simulink model "SiL_gram"  (R2025b)
settings: Solver=ode2  StartTime=0.0  StopTime=t_end  FixedStep=1/400  RelTol=1e-3
PreLoadFcn:
  | stepsize_sim = evalin('base', get_param(bdroot, 'FixedStep'));
undefined symbols (not defined in the file or in its folder): defaultConsts, defaultWP, DiscIntNeverNeededParam, dspblkCoreblockFVToolHelper, gcbh, navConsts, sensors, stepsize_ctrl
libraries: simulink x7, sharedutil x1, sharedtransform x1, aerolibanimutils x1
(part 3 of 3)

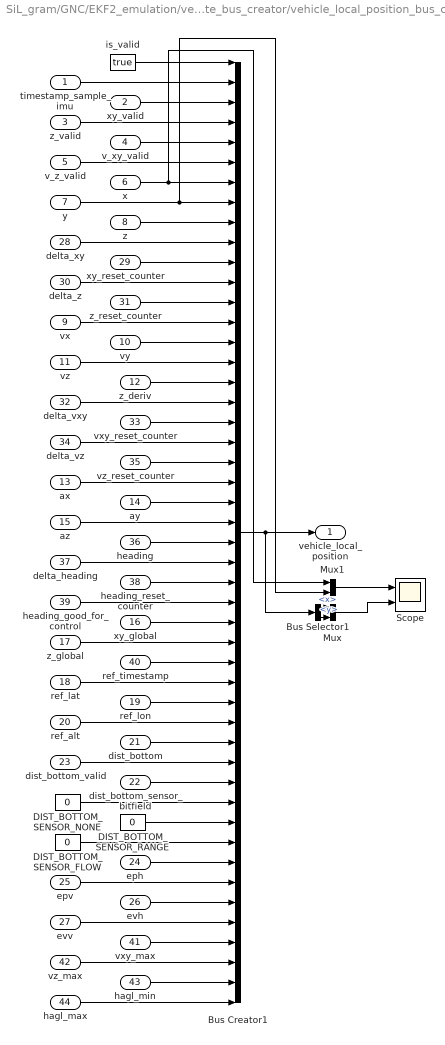
== system SiL_gram/GNC/EKF2_emulation/vehicle_state_bus_creator/vehicle_local_position_bus_creator ==
  timestamp_sample_imu : Inport
  xy_valid : Inport  Port=2  OutDataTypeStr=boolean  PortDimensions=1
  z_valid : Inport  Port=3  OutDataTypeStr=boolean  PortDimensions=1
  v_xy_valid : Inport  Port=4  OutDataTypeStr=boolean  PortDimensions=1
  v_z_valid : Inport  Port=5  OutDataTypeStr=boolean  PortDimensions=1
  x : Inport  Port=6  OutDataTypeStr=single  PortDimensions=1
  y : Inport  Port=7  OutDataTypeStr=single  PortDimensions=1
  z : Inport  Port=8  OutDataTypeStr=single  PortDimensions=1
  vx : Inport  Port=9  OutDataTypeStr=single  PortDimensions=1
  vy : Inport  Port=10  OutDataTypeStr=single  PortDimensions=1
  vz : Inport  Port=11  OutDataTypeStr=single  PortDimensions=1
  z_deriv : Inport  Port=12  OutDataTypeStr=single  PortDimensions=1
  ax : Inport  Port=13  OutDataTypeStr=single  PortDimensions=1
  ay : Inport  Port=14  OutDataTypeStr=single  PortDimensions=1
  az : Inport  Port=15  OutDataTypeStr=single  PortDimensions=1
  xy_global : Inport  Port=16  OutDataTypeStr=boolean  PortDimensions=1
  z_global : Inport  Port=17  OutDataTypeStr=boolean  PortDimensions=1
  ref_lat : Inport  Port=18  OutDataTypeStr=double  PortDimensions=1
  ref_lon : Inport  Port=19  OutDataTypeStr=double  PortDimensions=1
  ref_alt : Inport  Port=20  OutDataTypeStr=single  PortDimensions=1
  dist_bottom : Inport  Port=21  OutDataTypeStr=single  PortDimensions=1
  dist_bottom_sensor_bitfield : Inport  Port=22  OutDataTypeStr=uint8  PortDimensions=1
  dist_bottom_valid : Inport  Port=23  OutDataTypeStr=boolean  PortDimensions=1
  eph : Inport  Port=24  OutDataTypeStr=single  PortDimensions=1
  epv : Inport  Port=25  OutDataTypeStr=single  PortDimensions=1
  evh : Inport  Port=26  OutDataTypeStr=single  PortDimensions=1
  evv : Inport  Port=27  OutDataTypeStr=single  PortDimensions=1
  delta_xy : Inport  Port=28  OutDataTypeStr=single  PortDimensions=2
  xy_reset_counter : Inport  Port=29  OutDataTypeStr=uint8  PortDimensions=1
  delta_z : Inport  Port=30  OutDataTypeStr=single  PortDimensions=1
  z_reset_counter : Inport  Port=31  OutDataTypeStr=uint8  PortDimensions=1
  delta_vxy : Inport  Port=32  OutDataTypeStr=single  PortDimensions=2
  vxy_reset_counter : Inport  Port=33  OutDataTypeStr=uint8  PortDimensions=1
  delta_vz : Inport  Port=34  OutDataTypeStr=single  PortDimensions=1
  vz_reset_counter : Inport  Port=35  OutDataTypeStr=uint8  PortDimensions=1
  heading : Inport  Port=36  OutDataTypeStr=single  PortDimensions=1
  delta_heading : Inport  Port=37  OutDataTypeStr=single  PortDimensions=1
  heading_reset_counter : Inport  Port=38  OutDataTypeStr=uint8  PortDimensions=1
  heading_good_for_control : Inport  Port=39  OutDataTypeStr=boolean  PortDimensions=1
  ref_timestamp : Inport  Port=40  OutDataTypeStr=double  PortDimensions=1
  vxy_max : Inport  Port=41  OutDataTypeStr=single  PortDimensions=1
  vz_max : Inport  Port=42  OutDataTypeStr=single  PortDimensions=1
  hagl_min : Inport  Port=43  OutDataTypeStr=single  PortDimensions=1
  hagl_max : Inport  Port=44  OutDataTypeStr=single  PortDimensions=1
  Bus Selector1 : BusSelector  OutputSignals=x,y
  Bus Creator1 : BusCreator  Inputs=48  OutDataTypeStr=Bus: vehicle_local_position_bus
      settings: InheritFromInputs=off
  DIST_BOTTOM_SENSOR_FLOW : Constant  Value=0  OutDataTypeStr=uint8
  DIST_BOTTOM_SENSOR_NONE : Constant  Value=0  OutDataTypeStr=uint8
  DIST_BOTTOM_SENSOR_RANGE : Constant  Value=0  OutDataTypeStr=uint8
  Mux : Mux  Inputs=2
  Mux1 : Mux  Inputs=2
  Scope : Scope  NumInputPorts=2
      settings: ActiveDisplayYMinimum=-586.90811681747437  ActiveDisplayYMaximum=109.35261678695677  DataLoggingVariableName=ScopeData7
  is_valid : Constant  Value=true  OutDataTypeStr=boolean
  vehicle_local_position : Outport  OutDataTypeStr=Bus: vehicle_local_position_bus  VectorParamsAs1DForOutWhenUnconnected=off
  wires:
  is_valid/1 -> Bus Creator1/1
  xy_valid/1 -> Bus Creator1/3
  z_valid/1 -> Bus Creator1/4
  v_xy_valid/1 -> Bus Creator1/5
  v_z_valid/1 -> Bus Creator1/6
  x/1 -> Mux1/1, Bus Creator1/7
  y/1 -> Mux1/2, Bus Creator1/8
  z/1 -> Bus Creator1/9
  delta_xy/1 -> Bus Creator1/10
  xy_reset_counter/1 -> Bus Creator1/11
  delta_z/1 -> Bus Creator1/12
  z_reset_counter/1 -> Bus Creator1/13
  vx/1 -> Bus Creator1/14
  vy/1 -> Bus Creator1/15
  vz/1 -> Bus Creator1/16
  z_deriv/1 -> Bus Creator1/17
  delta_vxy/1 -> Bus Creator1/18
  vxy_reset_counter/1 -> Bus Creator1/19
  delta_vz/1 -> Bus Creator1/20
  vz_reset_counter/1 -> Bus Creator1/21
  ax/1 -> Bus Creator1/22
  ay/1 -> Bus Creator1/23
  az/1 -> Bus Creator1/24
  heading/1 -> Bus Creator1/25
  xy_global/1 -> Bus Creator1/29
  z_global/1 -> Bus Creator1/30
  ref_timestamp/1 -> Bus Creator1/31
  ref_lat/1 -> Bus Creator1/32
  ref_lon/1 -> Bus Creator1/33
  ref_alt/1 -> Bus Creator1/34
  dist_bottom/1 -> Bus Creator1/35
  dist_bottom_sensor_bitfield/1 -> Bus Creator1/37
  dist_bottom_valid/1 -> Bus Creator1/36
  eph/1 -> Bus Creator1/41
  epv/1 -> Bus Creator1/42
  evh/1 -> Bus Creator1/43
  evv/1 -> Bus Creator1/44
  vxy_max/1 -> Bus Creator1/45
  vz_max/1 -> Bus Creator1/46
  hagl_min/1 -> Bus Creator1/47
  hagl_max/1 -> Bus Creator1/48
  Bus Creator1/1 -> Bus Selector1/1, vehicle_local_position/1
  timestamp_sample_imu/1 -> Bus Creator1/2
  heading_good_for_control/1 -> Bus Creator1/28
  heading_reset_counter/1 -> Bus Creator1/27
  delta_heading/1 -> Bus Creator1/26
  DIST_BOTTOM_SENSOR_NONE/1 -> Bus Creator1/38
  DIST_BOTTOM_SENSOR_FLOW/1 -> Bus Creator1/40
  DIST_BOTTOM_SENSOR_RANGE/1 -> Bus Creator1/39
  Bus Selector1/1 -> Mux/1  "<x>"
  Bus Selector1/2 -> Mux/2  "<y>"
  Mux/1 -> Scope/2
  Mux1/1 -> Scope/1

== system SiL_gram/GNC/mavlink_receiver.cpp/GPS/Subsystem ==
  n : Inport
  e : Inport  Port=2
  d : Inport  Port=3
  Sqrt : Sqrt
  Square : Math  Operator=square
  Square1 : Math  Operator=square
  Square2 : Math  Operator=square
  Sum : Sum  Inputs=+++
  Out1 : Outport
  wires:
  Sqrt/1 -> Out1/1
  Sum/1 -> Sqrt/1
  n/1 -> Square/1
  Square/1 -> Sum/1
  d/1 -> Square2/1
  e/1 -> Square1/1
  Square1/1 -> Sum/2
  Square2/1 -> Sum/3

== system SiL_gram/GNC/mavlink_receiver.cpp/Waypoints/switch WPs ==
  Constant : Constant  Value=defaultWP.flightplan
  Manual Switch : ManualSwitch  CurrentSetting=0
  Terminator : Terminator
  landing WP : MATLAB Function  TreatAsAtomicUnit=on
  new flightplan : MATLAB Function  TreatAsAtomicUnit=on
  original : Outport
  modified : Outport  Port=2
  wires:
  new flightplan/1(flt_new) -> Manual Switch/1
  Constant/1 -> original/1, Manual Switch/2, new flightplan/1(fltplan)
  Manual Switch/1 -> modified/1
  landing WP/1(flt_new) -> Terminator/1

== matlab function SiL_gram/GNC/EKF2_emulation/MATLAB Function ==
  data: quat input single; eul_rad output single
function eul_rad=quat2euler(quat)

eul_rad = single([0;0;0]);
ysqr = quat(3) * quat(3);

t0 = 2 * (quat(1) * quat(2) + quat(3) * quat(4));
t1 = 1 - 2 * (quat(2) * quat(2) + ysqr);
eul_rad(1) = atan2(t0, t1);

t2 = 2 * (quat(1) * quat(3) - quat(4) * quat(2));
if t2 > 1
    t2 = single(1);
elseif t2 < -1
    t2 = -single(1);
end
eul_rad(2) = asin(t2);

t3 = 2 * (quat(1) * quat(4) + quat(2) * quat(3));
t4 = 1 - 2 * (ysqr + quat(4) * quat(4));
eul_rad(3) = atan2(t3, t4);

end

== matlab function SiL_gram/GNC/EKF2_emulation/MATLAB Function1 ==
  data: baro_rel input Bus: ifr_baro; h_ref input; ref_pos input; ref_valid input; baro_abs output Bus: ifr_baro
function baro_abs  = fcn(baro_rel,h_ref,ref_pos,ref_valid)

baro_abs.isValid = baro_rel.isValid;

if ref_valid
    baro_abs.height  = baro_rel.height + single(ref_pos(3)*1e-3);
else
    baro_abs.height  = baro_rel.height + h_ref;
end

end

== matlab function SiL_gram/GNC/mavlink_receiver.cpp/ifr_imu_filter.cpp/filterAccelMeasurementSecondOrder ==
  data: ome input; y output; zet input; acc input; stepsize_sim parameter
function y = fcn(ome,zet,acc,stepsize_sim)
persistent ykm1 ykm2 ukm1 ukm2

if isempty(ykm1)
    ykm1 = zeros(3,1,'single');
    ykm2 = zeros(3,1,'single');
    ukm1 = zeros(3,1,'single');
    ukm2 = zeros(3,1,'single');
end

subs1 = zet*ome*stepsize_sim;
subs2 = ome^2*stepsize_sim^2;

num = ykm2*(4*subs1-subs2-4) + ykm1*(8-2*subs2) + (ukm2+2*ukm1+acc)*subs2;
den = (4*subs1+subs2+4);

yk = num/den;
ukm2 = ukm1;
ukm1 = acc;
ykm2 = ykm1;
ykm1 = yk;

y = yk;

== matlab function SiL_gram/GNC/mavlink_receiver.cpp/Waypoints/switch WPs/new flightplan ==
  data: fltplan input; flt_new output
function flt_new = fcn(fltplan)

flt_new = fltplan;
flt_new(1,1)=5;
flt_new(6,:)=[-400,150,-100];
%flt_new(:,2)=flt_new(:,2)+200;
flt_new(:,3)=flt_new(:,3)-60;
flt_new(5,3)=flt_new(5,3)+20;

== matlab function SiL_gram/Sensors/ifr_imu_filter.cpp/MATLAB Function ==
  data: filt_num output single; filt_den output single; zeta input single; diff_num output single; diff_den output single; omega input single
function [filt_num,filt_den,diff_num,diff_den]  = tbv(zeta,omega)

T = single(0.01);
w = omega;
z = zeta;

scale = T^2*w^2+4*T*w*z+4;

%Discrete time IMU derivative and second order washout filter transfer function. See filter_design.m for more details.
diff_num = [2*T*w^2 0 -2*T*w^2]/scale;
diff_den = [T^2*w^2+4*T*w*z+4 2*T^2*w^2-8 T^2*w^2-4*T*w*z+4]/scale;

%Discrete time second order washout filter to synchronize phase shift between IMU derivative and actuator position signals. See filter_design.m for more details.
filt_num = [T^2*w^2, 2*T^2*w^2, T^2*w^2]/scale;
filt_den = [T^2*w^2+4*T*w*z+4 2*T^2*w^2-8 T^2*w^2-4*T*w*z+4]/scale;

== matlab function SiL_gram/GNC/mavlink_receiver.cpp/Waypoints/switch WPs/landing WP ==
  data: flt_new output
function flt_new = fcn()

flt_new = zeros(21,3);
flt_new(1,1)=1;
flt_new(2,:)=[100,0,0];

== matlab function SiL_gram/GNC/mavlink_receiver.cpp/ifr_imu_filter.cpp/MATLAB Function ==
  data: filt_num output single; filt_den output single; zeta input single; diff_num output single; diff_den output single; omega input single
function [filt_num,filt_den,diff_num,diff_den]  = tbv(zeta,omega)

T = single(0.01);
w = omega;
z = zeta;

scale = T^2*w^2+4*T*w*z+4;

%Discrete time IMU derivative and second order washout filter transfer function. See filter_design.m for more details.
diff_num = [2*T*w^2 0 -2*T*w^2]/scale;
diff_den = [T^2*w^2+4*T*w*z+4 2*T^2*w^2-8 T^2*w^2-4*T*w*z+4]/scale;

%Discrete time second order washout filter to synchronize phase shift between IMU derivative and actuator position signals. See filter_design.m for more details.
filt_num = [T^2*w^2, 2*T^2*w^2, T^2*w^2]/scale;
filt_den = [T^2*w^2+4*T*w*z+4 2*T^2*w^2-8 T^2*w^2-4*T*w*z+4]/scale;

== matlab function SiL_gram/GNC/mavlink_receiver.cpp/ifr_imu_filter.cpp/filterGyroMeasurementSecondOrder ==
  data: ome input; y output; zet input; rte input; stepsize_sim parameter
function y = fcn(ome,zet,rte,stepsize_sim)
persistent ykm1 ykm2 ukm1 ukm2

if isempty(ykm1)
    ykm1 = zeros(3,1,'single');
    ykm2 = zeros(3,1,'single');
    ukm1 = zeros(3,1,'single');
    ukm2 = zeros(3,1,'single');
end

subs1 = zet*ome*stepsize_sim;
subs2 = ome^2*stepsize_sim^2;

num = ykm2*(4*subs1-subs2-4) + ykm1*(8-2*subs2) + (ukm2+2*ukm1+rte)*subs2;
den = (4*subs1+subs2+4);

yk = num/den;
ukm2 = ukm1;
ukm1 = rte;
ykm2 = ykm1;
ykm1 = yk;

y = yk;

== matlab function SiL_gram/GNC/mavlink_receiver.cpp/ifr_imu_filter.cpp/filterGyroDerivativeSecondOrder ==
  data: ome input; y output; zet input; rte input; stepsize_sim parameter
function y = fcn(ome,zet,rte,stepsize_sim)
persistent ykm1 ykm2 ukm1 ukm2

if isempty(ykm1)
    ykm1 = zeros(3,1,'single');
    ykm2 = zeros(3,1,'single');
    ukm1 = zeros(3,1,'single');
    ukm2 = zeros(3,1,'single');
end

subs1 = zet*ome*stepsize_sim;
subs2 = ome^2*stepsize_sim^2;

num = ykm2*(4*subs1-subs2-4) + ykm1*(8-2*subs2) + 2*(rte-ukm2)*ome^2*stepsize_sim;
den = (4*subs1+subs2+4);

yk = num/den;
ukm2 = ukm1;
ukm1 = rte;
ykm2 = ykm1;
ykm1 = yk;

y = yk;

== matlab function SiL_gram/Sensors/ifr_imu_filter.cpp/filterAccelMeasurementSecondOrder ==
  data: ome input; y output; zet input; acc input; stepsize_sim parameter
function y = fcn(ome,zet,acc,stepsize_sim)
persistent ykm1 ykm2 ukm1 ukm2

if isempty(ykm1)
    ykm1 = zeros(3,1,'single');
    ykm2 = zeros(3,1,'single');
    ukm1 = zeros(3,1,'single');
    ukm2 = zeros(3,1,'single');
end

subs1 = zet*ome*stepsize_sim;
subs2 = ome^2*stepsize_sim^2;

num = ykm2*(4*subs1-subs2-4) + ykm1*(8-2*subs2) + (ukm2+2*ukm1+acc)*subs2;
den = (4*subs1+subs2+4);

yk = num/den;
ukm2 = ukm1;
ukm1 = acc;
ykm2 = ykm1;
ykm1 = yk;

y = yk;

== matlab function SiL_gram/Sensors/ifr_imu_filter.cpp/filterGyroDerivativeSecondOrder ==
  data: ome input; y output; zet input; rte input; stepsize_sim parameter
function y = fcn(ome,zet,rte,stepsize_sim)
persistent ykm1 ykm2 ukm1 ukm2

if isempty(ykm1)
    ykm1 = zeros(3,1,'single');
    ykm2 = zeros(3,1,'single');
    ukm1 = zeros(3,1,'single');
    ukm2 = zeros(3,1,'single');
end

subs1 = zet*ome*stepsize_sim;
subs2 = ome^2*stepsize_sim^2;

num = ykm2*(4*subs1-subs2-4) + ykm1*(8-2*subs2) + 2*(rte-ukm2)*ome^2*stepsize_sim;
den = (4*subs1+subs2+4);

yk = num/den;
ukm2 = ukm1;
ukm1 = rte;
ykm2 = ykm1;
ykm1 = yk;

y = yk;

== matlab function SiL_gram/Sensors/ifr_imu_filter.cpp/filterGyroMeasurementSecondOrder ==
  data: ome input; y output; zet input; rte input; stepsize_sim parameter
function y = fcn(ome,zet,rte,stepsize_sim)
persistent ykm1 ykm2 ukm1 ukm2

if isempty(ykm1)
    ykm1 = zeros(3,1,'single');
    ykm2 = zeros(3,1,'single');
    ukm1 = zeros(3,1,'single');
    ukm2 = zeros(3,1,'single');
end

subs1 = zet*ome*stepsize_sim;
subs2 = ome^2*stepsize_sim^2;

num = ykm2*(4*subs1-subs2-4) + ykm1*(8-2*subs2) + (ukm2+2*ukm1+rte)*subs2;
den = (4*subs1+subs2+4);

yk = num/den;
ukm2 = ukm1;
ukm1 = rte;
ykm2 = ykm1;
ykm1 = yk;

y = yk;

== matlab function SiL_gram/GNC/mavlink_receiver.cpp/Waypoints/MATLAB Function2 ==
  data: refPos input; llh2ned input; flightplan input; wp_lla output Bus: waypoint_list_bus
function wp_lla = mat2bus(refPos,llh2ned, flightplan)

wp_lla.is_valid = true;
wp_lla.lat = (single(refPos(1))+flightplan(2:end,1)/llh2ned(1))/1e7; %north
wp_lla.lon = (single(refPos(2))+flightplan(2:end,2)/llh2ned(2))/1e7; %east
wp_lla.alt = flightplan(2:end,3)/llh2ned(3)/1e3; %down
wp_lla.count = uint16(flightplan(1,1));

end

== matlab function SiL_gram/Sensors/ifr_imu_filter.cpp/IMU/Placement outside COG ==
  data: omega input; centrifugal_acc output; lever input; dwdt input
function centrifugal_acc = fcn(omega, lever, dwdt)

%centrifugal acceleration is -omega x(omega x lever)
centrifugal_acc = zeros(3,1);
centrifugal_acc = cross(omega,cross(omega,lever)) + cross(dwdt, lever);

== matlab function SiL_gram/GNC/EKF2_emulation/MATLAB Function8 ==
  data: gyro_raw input Bus: sensor_gyro_bus; gyro_m output; acc_raw input Bus: sensor_accel_bus; acc_m output; imu_filter input Bus: ifr_imu_filtered_bus; param input Bus: nav_parameterBus
function [gyro_m,acc_m] = fcn(gyro_raw,acc_raw,imu_filter,param)
pix_orientation = [param.pix_roll;param.pix_pitch;param.pix_yaw];

T1 = [1 0 0;0 cos(pix_orientation(1)) sin(pix_orientation(1));0 -sin(pix_orientation(1)) cos(pix_orientation(1))];
T2 = [cos(pix_orientation(2)) 0 -sin(pix_orientation(2));0 1 0;sin(pix_orientation(2)) 0 cos(pix_orientation(2))];
T3 = [cos(pix_orientation(3)) sin(pix_orientation(3)) 0;-sin(pix_orientation(3)) cos(pix_orientation(3)) 0;0 0 1];
T = T1*T2*T3;

if isequal(param.imu_filt.use_acc,single(1))
    acc_m = imu_filter.acc_filt;
else
    acc_m = T*[acc_raw.x;acc_raw.y;acc_raw.z];
end

if isequal(param.imu_filt.use_rte,single(1))
    gyro_m = imu_filter.rates_filt;
else
    gyro_m = T*[gyro_raw.x;gyro_raw.y;gyro_raw.z];
end

== matlab function SiL_gram/Remote_Control/MATLAB Function ==
  data: cur input; prev input; val input; y output
function y = add(cur,prev,val)

if isequal(prev,0)
    y = val + cur;
else
    y = val;
end

== matlab function SiL_gram/Remote_Control/MATLAB Function1 ==
  data: cur input; prev input; val input; y output
function y = add(cur,prev,val)

if isequal(prev,0)
    y = val + cur;
else
    y = val;
end

== matlab function SiL_gram/GNC/EKF2_emulation/acc transformation4 ==
  data: acc_b input; euler input; acc_g output; navConsts parameter Bus: nav_constantsBus
function acc_g  = acc_transform(acc_b,euler,navConsts)

tf3 = [cos(-euler(3)) sin(-euler(3)) 0; -sin(-euler(3)) cos(-euler(3)) 0; 0 0 1];
tf2 = [cos(-euler(2)) 0 -sin(-euler(2)); 0 1 0; sin(-euler(2)) 0 cos(-euler(2))];
tf1 = [1 0 0; 0 cos(-euler(1)) sin(-euler(1)); 0 -sin(-euler(1)) cos(-euler(1))];

acc_g = tf3*tf2*tf1*(acc_b)+[0;0;navConsts.g];

== matlab function SiL_gram/GNC/EKF2_emulation/barometer preprocessor ==
  settings: updateMethod=DISCRETE
  data: rawBaroData input Bus: sensor_baro_bus size=1; analysisParams output; height output; params input Bus: nav_parameterBus size=1; fixReference input boolean size=1; baro_rel output Bus: ifr_baro size=1; height_ref output; navConsts parameter
function [analysisParams,height,baro_rel,height_ref] = preprocessBaro(rawBaroData,params,fixReference,navConsts)
persistent refHeight_dyn fixed
if params.dynRefHeight
    loopIdentifier = single(1);
    if isempty(refHeight_dyn)
        refHeight_dyn = single(navConsts.initialPositionLla(3));
        fixed=false;
        loopIdentifier = single(10);
    end
    if isempty(fixed)
        fixed=false;
        loopIdentifier = loopIdentifier+single(100);
    end
    
    baro_rel.isValid=(rawBaroData.is_valid && rawBaroData.pressure>500);
    height=computeHeightFromPressure(rawBaroData.pressure, navConsts);
    if ~fixed
        loopIdentifier = loopIdentifier+single(1000);
        baro_rel.height=single(0);
        if fixReference
            fixed=true;
        else
            if navConsts.airStart %air start in simulation
            else
                refHeight_dyn = refHeight_dyn+params.biasSmoothingGain*(height-refHeight_dyn);
                loopIdentifier = loopIdentifier+single(10000);
            end
        end
    else
        baro_rel.height=height-refHeight_dyn;
        %baro.height=height;
    end
    height_ref = refHeight_dyn;
else
    loopIdentifier = single(0);
    refHeight_stat = params.referenceHeight;
    baro_rel.isValid=(rawBaroData.is_valid && rawBaroData.pressure>500);
    height=computeHeightFromPressure(rawBaroData.pressure, navConsts);
    if fixReference
        baro_rel.height=single(0);
    else
        baro_rel.height=height-refHeight_stat;
        %baro.height=height;
    end
    height_ref = refHeight_stat;
end
analysisParams = [navConsts.initialPositionLla(3),height,height_ref,loopIdentifier];
end

function height=computeHeightFromPressure(pressure, constants)
height=constants.referenceTemperature/constants.temperatureGradient*(1-(pressure/constants.referencePressure)^((constants.atmosphereKappa-1)/constants.atmosphereKappa));
end

== matlab function SiL_gram/GNC/EKF2_emulation/delay compensation ==
  data: translation input single size=6; position output single size=3; attitude output single size=4; rotation input single size=4; delRot input single size=4; delPos input single size=3; delVel input single size=3; delAtt input single size=4; velocity output single size=3; navConsts parameter size=1
function [position, attitude, velocity] = fcn(translation,rotation,delRot,delPos,delVel,delAtt,navConsts)
    timeDelay=navConsts.filterDelay;
    
    geoToRef=quaternionProduct(delAtt, [delRot(1); -delRot(2:4)]);
    refToGeoMat=quatToMat(geoToRef)';
    position=delPos+timeDelay*delVel+refToGeoMat*translation(1:3)+0.5*timeDelay^2*[0; 0; navConsts.g];
    velocity=delVel+refToGeoMat*translation(4:6)+timeDelay*[0; 0; navConsts.g];
    attitude=quaternionProduct(geoToRef, rotation);
end

function prod=quaternionProduct(q, p)
    [q0, qVec, p0, pVec]=deal(q(1), q(2:4), p(1), p(2:4));
    prod=[q0*p0-qVec'*pVec; q0*pVec+p0*qVec+cross(qVec, pVec)];
end

function mat=quatToMat(quat)
    [q0, q1, q2, q3]=deal(quat(1), quat(2), quat(3), quat(4));
    mat=[1-2*(q2^2+q3^2), 2*(q1*q2+q3*q0), 2*(q1*q3-q2*q0); ...
         2*(q1*q2-q3*q0), 1-2*(q1^2+q3^2), 2*(q2*q3+q1*q0); ...
         2*(q1*q3+q2*q0), 2*(q2*q3-q1*q0), 1-2*(q1^2+q2^2)];
end

== matlab function SiL_gram/Remote_Control/MATLAB Function2 ==
  data: cur input; prev input; val input; y output
function y = add(cur,prev,val)

if isequal(prev,0)
    y = val + cur;
else
    y = val;
end

== matlab function SiL_gram/Remote_Control/MATLAB Function3 ==
  data: cur input; prev input; val input; y output
function y = add(cur,prev,val)

if isequal(prev,0)
    y = val + cur;
else
    y = val;
end

== stateflow chart SiL_gram/Remote_Control/Mode Management  ==
  settings: updateMethod=DISCRETE  sampleTime=0.01
  state PIC
    en, du:
    mode_switch = 1;
    guidance_mode = -1;
    controller_mode = -1;
  state Takeoff_Loiter
    en, du:
    mode_switch = 0;
    guidance_mode = 0;
    controller_mode = 2;
  state Taxi
    en, du:
    mode_switch = 0;
    guidance_mode = -1;
    controller_mode = 1;
  state Landing
    en, du:
    mode_switch = -1;
    guidance_mode = 0;
    controller_mode = 3;
  (default) -> PIC
  PIC -> Landing [order 2] : [LDG>0]
  PIC -> Taxi [order 3] : [Taxi>0 && TO<1 && LDG<1]
  Landing -> PIC : [LDG<1]
  Taxi -> PIC [order 2] : [Taxi<1]
  PIC -> Takeoff_Loiter [order 1] : [TO>0 && LDG<1]
  Takeoff_Loiter -> PIC [order 1] : [TO<1]
  Taxi -> Takeoff_Loiter [order 1] : [TO>0 && LDG<1]
  Takeoff_Loiter -> Landing [order 2] : [LDG>0]
  Taxi -> Landing [order 3] : [LDG>0]
  data: mode_switch output; guidance_mode output; controller_mode output; Taxi input; LDG input; TO input

== matlab function SiL_gram/GNC/EKF2_emulation/gps preprocessor ==
  settings: updateMethod=DISCRETE
  data: geodeticReference output Bus: ifr_geodeticReference size=1; parameters input Bus: nav_parameterBus size=1; fixReference input; rawGpsData input Bus: vehicle_gps_position_bus size=1; gps output Bus: ifr_gps size=1; navConsts parameter size=1
function [geodeticReference,gps] =preprocessGps(parameters,fixReference,rawGpsData,navConsts)
persistent refPosValid refPosLlhRaw refLlhRawToNed earthMagneticField gravity isInitialized buffer counter
MAX_BUF_SIZE = 200;

if isempty(refPosLlhRaw)
    refPosLlhRaw = int32([navConsts.initialPositionLla(1:2)*1e7; navConsts.initialPositionLla(3)*1e3]);
    refPosValid = false;
    [refLlhRawToNed, earthMagneticField, gravity]=initialize(refPosLlhRaw, single(2020), navConsts);
    isInitialized=false;
    buffer = zeros(MAX_BUF_SIZE,3,'int32'); %Max 40s buffer
    counter = 1;
    %
end

bufferSize = parameters.gpsBufferTime * single(5);
gps.isValid=(rawGpsData.is_valid && rawGpsData.eph<=parameters.gpsAccuracyThreshold);

posLlhRaw=[rawGpsData.lat; rawGpsData.lon; rawGpsData.alt];

if ~isInitialized && gps.isValid
    gpsAvrg = zeros(1,3,'double');
    ctr = 0;
    if ~fixReference
        buffer(counter,:) = [rawGpsData.lat, rawGpsData.lon, rawGpsData.alt]; %update with new values
        if single(mod(counter,MAX_BUF_SIZE)) > bufferSize
            % bufferSize has to be converted from 'real32_T {aka float}' to 'real_T {aka double}' to match other operand of binary expression [-Werror=double-promotion]
            %determine average of gps values as reference
            for i = 0:bufferSize-1 %for loop equals sum(buffer(counter-bufferSize:counter,:))
                ctr = ctr + 1;
                gpsAvrg = gpsAvrg + double(buffer(counter-i,:));
            end
            refPos = int32(gpsAvrg'/ctr);
        else %mod(counter,MAX_BUF_SIZE) <= bufferSize
            %consider all previous elements of buffer matrix
            for i = 1:mod(counter,MAX_BUF_SIZE) %for loop equals sum(buffer(counter-bufferSize:counter,:))
                ctr = ctr + 1;
                gpsAvrg = gpsAvrg + double(buffer(i,:));
            end
            %consider all relevant elements at the end of buffer matrix
            for i = 1:bufferSize-mod(counter,MAX_BUF_SIZE) %for loop equals sum(buffer)'/sum(~all(buffer==0,2))
                currBuff = double(buffer(end+1-i,:));
                if ~isequal(currBuff,zeros(1,3))
                    ctr = ctr + 1;
                    gpsAvrg = gpsAvrg + currBuff;
                end
            end
            refPos = int32(gpsAvrg'/ctr);
        end
        if navConsts.airStart %air start in simulation
            refPosLlhRaw=refPos-int32([0*1e7; 0*1e7; navConsts.initialBaroReading*1e3]);
        else
            refPosLlhRaw=refPos;
        end
        if rawGpsData.time_utc_usec~=0
            year=single(1970)+single(rawGpsData.time_utc_usec/(365.24*24*3600*1.0e6));
        else
            year=single(2020);
        end
        [refLlhRawToNed, earthMagneticField, gravity]=initialize(refPosLlhRaw, year, navConsts);
        if counter >= MAX_BUF_SIZE
            counter = 1;
        else
            counter = counter + 1;
        end
    else
        isInitialized=true;
    end
    refPosValid = true;
end

gps.position=refLlhRawToNed.*single(posLlhRaw-[refPosLlhRaw(1:2);0]);
gps.velocity=[rawGpsData.vel_n_m_s; rawGpsData.vel_e_m_s; rawGpsData.vel_d_m_s];

geodeticReference.earthMagneticField = earthMagneticField;
geodeticReference.gravity =            gravity;
geodeticReference.refLlhRawToNed =     refLlhRawToNed;
geodeticReference.refPosLlhRaw =       refPosLlhRaw;
geodeticReference.refPosValid =        refPosValid;
end

function [llhRawToNed, magRefNed, gravity]=initialize(refLlhPosRaw, year, constants)
semiMajorAxis=single(6378137);
eccentricity=single(8.1819190842622e-2);
posScaleFactor=single([1e-7*pi/180; 1e-7*pi/180; 1e-3]);
lattitudeRef=posScaleFactor(1)*single(refLlhPosRaw(1)); %[rad]
longitudeRef=posScaleFactor(2)*single(refLlhPosRaw(2)); %[rad]
heightRef=posScaleFactor(3)*single(refLlhPosRaw(3)); %[m]
R0=semiMajorAxis/sqrt(1-eccentricity^2*sin(lattitudeRef)^2);
llhRawToNed=[(1-eccentricity^2)/semiMajorAxis^2*R0^3+heightRef; (R0+heightRef)*cos(lattitudeRef); -1].*posScaleFactor;

gamma=9.7803253359;
k=0.0019318526464;
dgdh=3.0877e-06;
ldgdh=4.50e-09;
gravity=single([0; 0; gamma*(1+k*sin(lattitudeRef)^2)/sqrt(1-eccentricity^2*sin(lattitudeRef)^2)-(dgdh-ldgdh*sin(lattitudeRef)^2)*heightRef]);
magRefNed=magnet([lattitudeRef; longitudeRef; heightRef], max(single(year-2000), single(0))*365, constants);
end

function magRefNED = magnet(llh, days, constants) % Inputs % r Geocentric radius % theta Latitude measured in degrees positive from equator % phi Longitude measured in degrees positive east from Greenwich % days Decimal days since January 1, 2000 % % Outputs - magnetic field strength in local tangential coordinates % Br B in radial direction % Bt B in theta direction % Bp B in phi direction
lat=pi/2-llh(1);
lon=llh(2);
a=6371200;
r=a+llh(3);
% Checks to see if located at either pole to avoid singularities
if (lat>single(-pi*1e-7) && lat<single(pi*1e-7))
    lat=single(pi*1e-7);
elseif(lat<single(pi*(1+1e-7)) && lat>single(pi*(1-1e-7)))
    lat=single(pi*(1-1e-7));
end

N=13;
g = constants.g0 + constants.dg*days/365.25;
h = constants.h0 + constants.dh*days/365.25;

[Br, Bt, Bp, dP11, dP10, P20, dP20]=deal(single(0));
[P10, P11]=deal(single(1));
[cosLat, sinLat]=deal(cos(lat), sin(lat));
for m=0:N
    for n=1:N
        if m<=n
            % Calculate Legendre polynomials and derivatives recursively
            if n==m
                P2 = sinLat*P11;
                dP2 = sinLat*dP11 + cosLat*P11;
                P11=P2; P10=P11; P20=single(0); dP11=dP2; dP10=dP11; dP20=single(0);
            elseif n==1
                P2 = cosLat*P10;
                dP2 = cosLat*dP10 - sinLat*P10;
                P20=P10; P10=P2; dP20=dP10; dP10=dP2;
            else
                K = ((n-1)^2-m^2)/((2*n-1)*(2*n-3));
                P2 = cosLat*P10 - K*P20;
                dP2 = cosLat*dP10 - sinLat*P10 - K*dP20;
                P20=P10; P10=P2; dP20=dP10; dP10=dP2;
            end
            Br = Br + (a/r)^(n+2)*(n+1)*((g(n,m+1)*cos(m*lon) + h(n,m+1)*sin(m*lon))*P2);
            Bt = Bt + (a/r)^(n+2)*((g(n,m+1)*cos(m*lon) + h(n,m+1)*sin(m*lon))*dP2);
            Bp = Bp + (a/r)^(n+2)*(m*(-g(n,m+1)*sin(m*lon) + h(n,m+1)*cos(m*lon))* P2);
        end
    end
end
magRefSphere = [Br;-Bt;-Bp/sinLat];
e = 0*pi/180;
magRefNED = [-sin(e),-cos(e),0;0,0,1;-cos(e),sin(e),0]*magRefSphere*10^-9;
end

== matlab function SiL_gram/GNC/EKF2_emulation/imu integration ==
  data: imu input Bus: ifr_imu size=1; translation output single size=6; rotation output single size=4; delayedImu input Bus: ifr_imu size=1; delayedRotation input single size=4; navConsts parameter size=1
function [translation, rotation] = integrateImu(imu, delayedImu, delayedRotation, navConsts)
    persistent quaternion x
    
    delayedImu.acceleration = delayedImu.acceleration;% + [0; 0; 9.81];
    imu.acceleration = imu.acceleration; %+ [0; 0; 9.81];
    dt=navConsts.stepSize;
    n=round(navConsts.filterDelay/dt);
    if isempty(quaternion)
        quaternion=single([1; 0; 0; 0]);
        x=zeros(6, 1, 'single');
    end
    rotation=quaternion;
    translation=x;
    
    I=eye(3, 'single');
    O=zeros(3, 'single');
    x=[I, dt*I; O, I]*x+[single(0.5)*dt^2*I, -dt^2*(n+single(0.5))*I; dt*I, -dt*I]*[quatToMat(rotation)'*imu.acceleration; quatToMat(delayedRotation)'*delayedImu.acceleration];
    quaternion=quaternion+single(0.5)*dt*[-imu.rate'*quaternion(2:4); imu.rate*quaternion(1)-cross(imu.rate, quaternion(2:4))];
    quaternion=quaternion/norm(quaternion);
end

function mat=quatToMat(quat)
    [q0, q1, q2, q3]=deal(quat(1), quat(2), quat(3), quat(4));
    mat=[1-2*(q2^2+q3^2), 2*(q1*q2+q3*q0), 2*(q1*q3-q2*q0); ...
         2*(q1*q2-q3*q0), 1-2*(q1^2+q3^2), 2*(q2*q3+q1*q0); ...
         2*(q1*q3+q2*q0), 2*(q2*q3-q1*q0), 1-2*(q1^2+q2^2)];
end

== matlab function SiL_gram/GNC/EKF2_emulation/imu preprocessor ==
  settings: updateMethod=DISCRETE
  data: time input single size=1; gyroBiasOut output; parameters input Bus: nav_parameterBus; fixGyroBias input boolean size=1; rateRaw input single size=3; imu output Bus: ifr_imu size=1; accRaw input single size=3
function [gyroBiasOut,imu]=preprocessImuData(time,parameters,fixGyroBias,rateRaw,accRaw)
persistent gyroBias fixed
if isempty(gyroBias)
    gyroBias=zeros(3, 1, 'single');
    fixed=false;
end

if ~fixGyroBias && ~fixed
    if isequal(parameters.imu_filt.use_rte,single(1)) %IMU filter module already uses gyro bias signal
        gyroBias=gyroBias+parameters.biasSmoothingGain*(rateRaw-gyroBias);
    end
else
    fixed=true;
end
imu.time=time;
imu.rate=rateRaw-gyroBias;
%imu.rate=rateRaw;
imu.acceleration= accRaw;
gyroBiasOut=gyroBias;
end

== matlab function SiL_gram/GNC/EKF2_emulation/magnetometer preprocessor ==
  data: vehicle_mag input Bus: vehicle_magnetometer_bus; mag output Bus: ifr_mag size=1
function mag=preprocessMagnetometer(vehicle_mag)
    mag.isValid=vehicle_mag.is_valid;
    mag.magneticField=1000.0*vehicle_mag.magnetometer_ga;
                                %single*(1e-4)
end

== matlab function SiL_gram/GNC/EKF2_emulation/navigation filter ==
  data: imu input Bus: ifr_imu size=1; z_valid output; para input Bus: nav_parameterBus size=1; pos output single size=3; baro input Bus: ifr_baro size=1; geoRef input Bus: ifr_geodeticReference; gps input Bus: ifr_gps size=1; mag input Bus: ifr_mag size=1; startFilter input boolean size=1; vel output single size=3; att output single size=4; navConsts parameter size=1; errVar output single size=9; sensors_valid output; mag_logger output Bus: navigation_mag_bus
function [z_valid,pos,vel,att,errVar,sensors_valid,mag_logger]=estimateVehicleState(imu,para,baro,geoRef,gps,mag,startFilter,navConsts)
persistent state covariance filterIsRunning timing

if isempty(state)
    state=[zeros(6, 1, 'single'); 1; zeros(3, 1, 'single')];
    covariance=diag(single([25, 25, 25, 4, 4, 4, 0.1, 0.1, 0.1]));
    filterIsRunning=false;
    timing=struct('sinceGps', para.gpsTimeout, 'lastTime', imu.time-navConsts.stepSize);
end

stepSize=imu.time-timing.lastTime;
timing.lastTime=imu.time;

if gps.isValid
    if timing.sinceGps>=para.gpsTimeout && filterIsRunning
        [state, covariance]=resetUsingGps(para, state, covariance, gps);
        gps.isValid=false;
    end
    timing.sinceGps=single(0);
else
    timing.sinceGps=timing.sinceGps+stepSize;
end

z_valid = timing.sinceGps<para.gpsTimeout;

if ~filterIsRunning
    if startFilter
        state(7:10)=initQuat(mag.magneticField, imu.acceleration);
        covariance(7:9, 7:9)=diag(single([0.1,0.1,0.1]));
        % next time GPS is available, horizontal position and velocity
        % shall be set to measurement rather than being updated
        [timing.sinceGps, filterIsRunning]=deal(para.gpsTimeout, true);
    end
    [pos, vel, att, errVar]=deal(state(1:3), state(4:6), state(7:10), diag(covariance));
    mag_logger.is_valid = false;
    mag_logger.state = zeros(10, 1, 'single');
    mag_logger.meas = zeros(3, 1, 'single');
    mag_logger.t = zeros(9, 1, 'single');
    mag_logger.ref = zeros(3, 1, 'single');
    mag_logger.residual = zeros(1, 1, 'single');
    mag_logger.h = zeros(9, 1, 'single');
    mag_logger.r = zeros(1, 1, 'single');
    mag_logger.gibbs_state = zeros(9, 1, 'single');
    mag_logger.attitude = zeros(3, 1, 'single');
else
    if timing.sinceGps<para.gpsTimeout
        [pos, vel, att, errVar, state, covariance, mag_logger]=runFilter(para, state, covariance, 1:9,...
            imu, stepSize, mag, gps, baro,geoRef);
    else
        [pos, vel, att, errVar, state, covariance, mag_logger]=runFilter(para, state, covariance, [3, 6:9],...
            imu, stepSize, mag, gps, baro,geoRef);
    end
end
sensors_valid = [mag.isValid;gps.isValid;baro.isValid];
end

function [position, velocity, attitude, errorVariances, state, covariance, mag_logger]=runFilter(parameters, state, covariance, subStateIndices, imu, stepSize,...
    mag, gps, baro,geoRef)
[state, covariance, mag_logger]=update(parameters, state, covariance, subStateIndices, mag, gps, baro, imu.acceleration,geoRef);
[position, velocity, attitude, errorVariances]=deal(state(1:3), state(4:6), state(7:10), diag(covariance));
[state, covariance]=predict(parameters, state, covariance, subStateIndices, imu, stepSize,geoRef.gravity);
end

function [state, covariance]=predict(parameters, state, covariance, iSub, imu, stepSize, g)
[v, q]=deal(state(4:6), state(7:10));

I=eye(3, 'single');
O=zeros(3, 'single');

bodyToGeo=quatToMat(q)';
stateIncrement=[stepSize*v+0.5*stepSize^2*(bodyToGeo*imu.acceleration+g);...
    stepSize*(bodyToGeo*imu.acceleration+g);...
    0.5*stepSize*[0, -imu.rate'; imu.rate, -skew(imu.rate)]*q];
F=[I, stepSize*I, -0.5*stepSize^2*bodyToGeo*skew(imu.acceleration);...
    O,          I,       -stepSize*bodyToGeo*skew(imu.acceleration);...
    O,          O,                        I-stepSize*skew(imu.rate)];
GQImuGT=[0.25*stepSize^4*parameters.sigmaAcc^2*I, 0.5*stepSize^3*parameters.sigmaAcc^2*I,                                         O;...
    0.5*stepSize^3*parameters.sigmaAcc^2*I,     stepSize^2*parameters.sigmaAcc^2*I,                                         O;...
    O,                                            O, stepSize^2*parameters.sigmaGyro^2*I];

covariance(iSub, iSub)=F(iSub, iSub)*covariance(iSub, iSub)*F(iSub, iSub)'+GQImuGT(iSub, iSub);
state([iSub, end])=state([iSub, end])+stateIncrement([iSub, end]);
state(7:10)=normalize(state(7:10));
end

function [state, covariance, mag_logger]=update(parameters, state, covariance, iSub, mag, gps, baro, acc, geoRef)
geoToBody=quatToMat(state(7:10));
bodyToGeo=geoToBody';
gibbsState=[state(1:6); zeros(3, 1, 'single')]; % expected attitude error (gibbs vector) is zero
if mag.isValid
    [residual_mag, H, R]=magMeasurementModel(parameters, mag.magneticField, bodyToGeo,geoRef.earthMagneticField);
    [gibbsState(iSub), covariance(iSub, iSub)]=performKalmanUpdate(gibbsState(iSub), covariance(iSub, iSub), residual_mag, H(:, iSub), R);
    mag_logger.is_valid = true;
    mag_logger.state = state;
    mag_logger.meas = mag.magneticField;
    mag_logger.t = reshape(bodyToGeo, [9 1]);
    mag_logger.ref = geoRef.earthMagneticField;
    mag_logger.residual = residual_mag;
    mag_logger.h = H';
    mag_logger.r = R;
    mag_logger.gibbs_state = gibbsState;
    mag_logger.attitude = zeros(3, 1, 'single');
else
    mag_logger.is_valid = false;
    mag_logger.state = zeros(10, 1, 'single');
    mag_logger.meas = zeros(3, 1, 'single');
    mag_logger.t = zeros(9, 1, 'single');
    mag_logger.ref = zeros(3, 1, 'single');
    mag_logger.residual = zeros(1, 1, 'single');
    mag_logger.h = zeros(9, 1, 'single');
    mag_logger.r = zeros(1, 1, 'single');
    mag_logger.gibbs_state = gibbsState;
    mag_logger.attitude = zeros(3, 1, 'single');
end
if gps.isValid
    [residual, H, R]=gpsMeasurementModel(parameters, gps.position, gps.velocity, gibbsState(1:3), gibbsState(4:6), geoRef.refPosLlhRaw);
    [gibbsState(iSub), covariance(iSub, iSub)]=performKalmanUpdate(gibbsState(iSub), covariance(iSub, iSub), residual, H(:, iSub), R);
elseif numel(iSub)<numel(gibbsState)-2 % only use acceleration update if neither GPS nor LOS rate are available
    [residual, H, R]=accMeasurementModel(parameters, acc, geoToBody, geoRef.gravity);
    [gibbsState(iSub), covariance(iSub, iSub)]=performKalmanUpdate(gibbsState(iSub), covariance(iSub, iSub), residual, H(:, iSub), R);
    gibbsState(4:5)=0.995*gibbsState(4:5); % velocity estimate is likely to be far off, hence it is damped
end
if baro.isValid
    [residual, H, R]=baroMeasurementModel(parameters, baro.height, -gibbsState(3));
    [gibbsState(iSub), covariance(iSub, iSub)]=performKalmanUpdate(gibbsState(iSub), covariance(iSub, iSub), residual, H(:, iSub), R);
end
state=[gibbsState(1:6); normalize(quaternionProduct(state(7:10), [2; gibbsState(7:9)]))];
end

function [residual_mag, measurementMatrix, measurementCovariance]=magMeasurementModel(parameters, mag, bodyToGeo, magGeoRef)
magGeo=bodyToGeo*mag;
measurementMatrix=[zeros(1, 6, 'single'), bodyToGeo(3, :)];
normProduct=norm(magGeoRef(1:2))*norm(magGeo(1:2));
denominator=normProduct+magGeoRef(1:2)'*magGeo(1:2);
epsilon=single(1e-3);
sigmaMag=single(1e-4)*parameters.sigmaMag; % unit should be T but is Gs
if denominator>epsilon*normProduct
    residual_mag=2*(magGeo(1)*magGeoRef(2)-magGeo(2)*magGeoRef(1))/denominator;
    measurementCovariance=(2*norm(magGeo(1:2))*sigmaMag/denominator)^2;
else % error is close to 180 deg, circumventing singularity...
    residual_mag=2*sqrt(2/epsilon-1);
    measurementCovariance=(2*sigmaMag/(epsilon*norm(magGeoRef(1:2))))^2;
end
end

function [residual, measurementMatrix, measurementCovariance]=gpsMeasurementModel(parameters, gpsPos, gpsVel, pos, vel, geoRef)
residual=[gpsPos-pos; gpsVel-vel];
measurementMatrix=[eye(6, 'single'), zeros(6, 3, 'single')];
measurementCovariance=diag([parameters.sigmaGpsPosXy*[1/cos(pi/180*1e-7*double(geoRef(1))); 1]; parameters.sigmaGpsPosZ;...
    parameters.sigmaGpsVelXy*[1/cos(pi/180*1e-7*double(geoRef(1))); 1]; parameters.sigmaGpsVelZ].^2);
end

function [residual, measurementMatrix, measurementCovariance]=baroMeasurementModel(parameters, baroHeight, height)
residual=baroHeight-height;
measurementMatrix=[zeros(1, 2, 'single'), -1, zeros(1, 6, 'single')];
measurementCovariance=parameters.sigmaBaro^2;
end

function [residual, measurementMatrix, measurementCovariance]=accMeasurementModel(parameters, acc, geoToBody, gravity)
residual=acc+geoToBody*gravity;
measurementMatrix=[zeros(3, 6, 'single'), -skew(geoToBody*gravity)];
measurementCovariance=parameters.sigmaAccelerationUpdate^2*eye(3, 'single');
end

function [state, covariance]=performKalmanUpdate(state, covariance, residual, H, R)
S=H*covariance*H'+R;
K=covariance*H'/S;
state=state+K*residual;
covariance=covariance-K*H*covariance;
end

function [state, covariance]=resetUsingGps(parameters, state, covariance, gps)
state(1:2)=gps.position(1:2);
covariance(1:2, 1:2)=parameters.sigmaGpsPosXy.^2*eye(2, 'single');
[covariance(1:2, 3:end), covariance(3:end, 1:2)]=deal(single(0));
state(4:6)=gps.velocity;
covariance(4:6, 4:6)=diag([parameters.sigmaGpsVelXy([1; 1]); parameters.sigmaGpsVelZ].^2);
[covariance(4:6, [1:3, 7:end]), covariance([1:3, 7:end], 4:6)]=deal(single(0));
end

function q=initQuat(magMeas, accMeas)
% geodetic axes in body frame using Gram-Schmidt process
basisZ=-normalize(accMeas);
basisX=normalize(magMeas-(magMeas'*basisZ)*basisZ);
q=matToQuat([basisX, cross(basisZ, basisX), basisZ]);
end

function n=normalize(v)
n=v./repmat(sqrt(sum(v.^2)), size(v, 1), 1);
end

function s=skew(v)
s=[     0, -v(3),  v(2);...
    v(3),     0, -v(1);...
    -v(2),  v(1),     0];
end

function prod=quaternionProduct(q, p)
[q0, qVec, p0, pVec]=deal(q(1), q(2:4), p(1), p(2:4));
prod=[q0*p0-qVec'*pVec; q0*pVec+p0*qVec+cross(qVec, pVec)];
end

function mat=quatToMat(quat)
[q0, q1, q2, q3]=deal(quat(1), quat(2), quat(3), quat(4));
mat=[1-2*(q2^2+q3^2), 2*(q1*q2+q3*q0), 2*(q1*q3-q2*q0); ...
    2*(q1*q2-q3*q0), 1-2*(q1^2+q3^2), 2*(q2*q3+q1*q0); ...
    2*(q1*q3+q2*q0), 2*(q2*q3-q1*q0), 1-2*(q1^2+q2^2)];
end

function quat=matToQuat(mat)
quat=zeros(4, 1, 'single');
tr=trace(mat);
if (tr>0)
    quat=[1+tr; mat(2, 3)-mat(3, 2); mat(3, 1)-mat(1, 3); mat(1, 2)-mat(2, 1)];
else
    [~, iMaxD]=max(diag(mat));
    switch iMaxD
        case 1, quat=[mat(2, 3)-mat(3, 2); 1+mat(1, 1)-mat(2, 2)-mat(3, 3); mat(1, 2)+mat(2, 1); mat(3, 1)+mat(1, 3)];
        case 2, quat=[mat(3, 1)-mat(1, 3); mat(1, 2)+mat(2, 1); 1-mat(1, 1)+mat(2, 2)-mat(3, 3); mat(2, 3)+mat(3, 2)];
        case 3, quat=[mat(1, 2)-mat(2, 1); mat(3, 1)+mat(1, 3); mat(2, 3)+mat(3, 2); 1-mat(1, 1)-mat(2, 2)+mat(3, 3)];
    end
end
quat=normalize(quat);
end

== matlab function SiL_gram/Sensors/Fault_Simulation/MATLAB Function ==
  data: p_mb input; ias output
function ias = BaroToIAS(p_mb)

p_Pa = p_mb * 100;

ias = sqrt(p_Pa*2/1.225);

== matlab function SiL_gram/Sensors/Fault_Simulation/MATLAB Function1 ==
  data: valid output; sensors parameter; defaultConsts parameter
function valid = lidar_valid(sensors,defaultConsts)
persistent counter

if isempty(counter)
    counter = 1;
end
if defaultConsts.sensorsReal
    if counter == 1
        valid = true;
    else
        valid = false;
    end
    counter = counter + 1;
    if counter > sensors.lidar.freq
        counter = 1;
    end
else
    valid = true;
end
end

== matlab function SiL_gram/Sensors/Fault_Simulation/MATLAB Function2 ==
  data: valid output; sensors parameter; defaultConsts parameter
function valid = gps_valid(sensors,defaultConsts)
persistent counter

if isempty(counter)
    counter = 1;
end
if defaultConsts.sensorsReal
    if counter == 1
        valid = true;
    else
        valid = false;
    end
    counter = counter + 1;
    if counter > sensors.gps.freq
        counter = 1;
    end
else
    valid = true;
end
end

== matlab function SiL_gram/Sensors/Fault_Simulation/MATLAB Function3 ==
  data: valid output; sensors parameter; defaultConsts parameter
function valid = mag_valid(sensors,defaultConsts)
persistent counter

if isempty(counter)
    counter = 1;
end
if defaultConsts.sensorsReal
    if counter == 1
        valid = true;
    else
        valid = false;
    end
    counter = counter + 1;
    if counter > sensors.mag.freq
        counter = 1;
    end
else
    valid = true;
end
end

== matlab function SiL_gram/Sensors/Fault_Simulation/MATLAB Function4 ==
  data: valid output boolean; sensors parameter; defaultConsts parameter
function valid = baro_valid(sensors,defaultConsts)
persistent counter

if isempty(counter)
    counter = 1;
end
if defaultConsts.sensorsReal
    if counter < sensors.airData.freq
        valid = false;
    elseif counter > sensors.airData.freq
        if rand(1,1) < 1/3
            valid = true;
        else
            valid = false;
        end
    else
        valid = true;
    end
    counter = counter + 1;
else
    valid = true;
end
end

== matlab function SiL_gram/GNC/mavlink_receiver.cpp/Waypoints/Geodetic Reference ==
  settings: updateMethod=DISCRETE
  data: refPos output; defaultConsts parameter size=1; llh2ned output
function [refPos,llh2ned]  =initialPosition_To_geodeticReference(defaultConsts)
persistent refPosLlhRaw refLlhRawToNed
if isempty(refPosLlhRaw)
    semiMajorAxis=single(6378137);
    eccentricity=single(8.1819190842622e-2);
    posScaleFactor=single([1e-7*pi/180; 1e-7*pi/180; 1e-3]);
    
    refPosLlhRaw = int32([defaultConsts.initialPositionLla(1:2)*1e7; defaultConsts.initialPositionLla(3)*1e3]);
    R0=semiMajorAxis/sqrt(1-eccentricity^2*sin(posScaleFactor(1)*single(refPosLlhRaw(1)))^2);
    refLlhRawToNed = [(1-eccentricity^2)/semiMajorAxis^2*R0^3+posScaleFactor(3)*single(refPosLlhRaw(3)); (R0+posScaleFactor(3)*single(refPosLlhRaw(3)))*cos(posScaleFactor(1)*single(refPosLlhRaw(1))); -1].*posScaleFactor;
end
refPos = refPosLlhRaw;
llh2ned = refLlhRawToNed;
end

== matlab function SiL_gram/GNC/mavlink_receiver.cpp/Baro/height2baro ==
  data: height input; pressure output; defaultConsts parameter
function pressure = HeightToBaro(height,defaultConsts)
    
    height_corrected = height+defaultConsts.initialPositionLla(3);
    
    pressure = defaultConsts.referencePressure*(1-height_corrected*defaultConsts.temperatureGradient/defaultConsts.referenceTemperature)^(defaultConsts.atmosphereKappa/(defaultConsts.atmosphereKappa-1)); %pressure in [Pa]
    
end
